simulink model "one"  (R2021a)
settings: Solver=VariableStepAuto  StartTime=0.0  StopTime=10.0  RelTol=1e-3
values from neighbouring files (symbols this model uses):
  A = eval(simplify(A))    [cfg_one.m]
  B = eval(simplify(B))    [cfg_one.m]
  K = acker(A, B, [-20 -20 -200])    [cfg_one.m]
  u_eq = double(solve(subs(fxu(1), x1, x1_eq(2))))    [cfg_one.m]
  x1_eq = double(x1_eq(2))    [cfg_one.m]
  x2_eq = 1    [cfg_one.m]
  x3_eq = 0    [cfg_one.m]
libraries: cstblocks x4
settings Model: Creator=Acer  LastModifiedBy=Acer

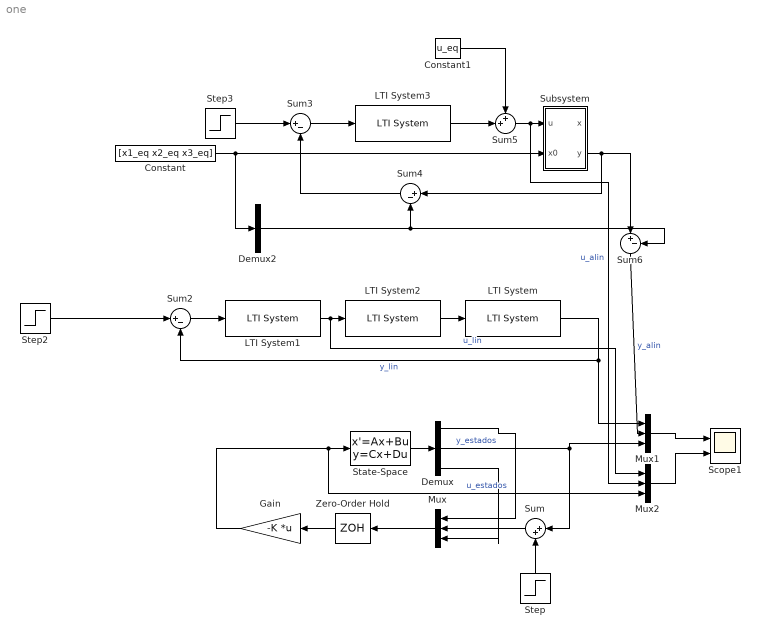
== system one ==
  Constant : Constant  Value=[x1_eq x2_eq x3_eq]
  Constant1 : Constant  Value=u_eq
  Demux : Demux  Outputs=3
  Demux2 : Demux  Outputs=3
  Gain : Gain  Gain=-K  Multiplication=Matrix(K*u) (u vector)
  LTI System : cstblocks/LTI System  sys=P  IC=[]
  LTI System1 : cstblocks/LTI System  sys=Contr  IC=[]
  LTI System2 : cstblocks/LTI System  sys=pade_raro  IC=[]
  LTI System3 : cstblocks/LTI System  sys=Contr  IC=[]
  Mux : Mux  Inputs=3
  Mux1 : Mux  Inputs=3
  Mux2 : Mux  Inputs=3
  Scope1 : Scope  NumInputPorts=2
  State-Space : StateSpace  A=A  B=B  C=eye(3)  D=zeros(3,1)  InitialCondition=0
  Step : Step  After=-0.01  SampleTime=0
  Step2 : Step  After=0.01  SampleTime=0
  Step3 : Step  After=0.01  SampleTime=0
  Subsystem : Subsystem
  Sum : Sum  Inputs=|++
  Sum{2..4,6} (4 alike) : Sum  Inputs=|+-
  Sum5 : Sum  Inputs=++|
  Zero-Order Hold : ZeroOrderHold  SampleTime=0.01/2
  wires:
  Gain/1 -> Mux2/3, State-Space/1  "u_estados"
  State-Space/1 -> Demux/1
  Demux/1 -> Mux/1
  Demux/2 -> Mux1/3, Sum/1  "y_estados"
  Demux/3 -> Mux/3
  Sum/1 -> Mux/2
  Step/1 -> Sum/2
  LTI System2/1 -> LTI System/1
  LTI System1/1 -> Mux2/1, LTI System2/1  "u_lin"
  Mux/1 -> Zero-Order Hold/1
  Zero-Order Hold/1 -> Gain/1
  LTI System/1 -> Mux1/1, Sum2/2  "y_lin"
  Sum2/1 -> LTI System1/1
  Step2/1 -> Sum2/1
  Subsystem/2(y) -> Sum6/1, Sum4/1
  Sum3/1 -> LTI System3/1
  Constant/1 -> Demux2/1, Subsystem/2(x0)
  Sum4/1 -> Sum3/2
  Demux2/2 -> Sum6/2, Sum4/2
  LTI System3/1 -> Sum5/2
  Sum5/1 -> Mux2/2, Subsystem/1(u)  "u_alin"
  Constant1/1 -> Sum5/1
  Step3/1 -> Sum3/1
  Sum6/1 -> Mux1/2  "y_alin"
  Mux1/1 -> Scope1/1
  Mux2/1 -> Scope1/2

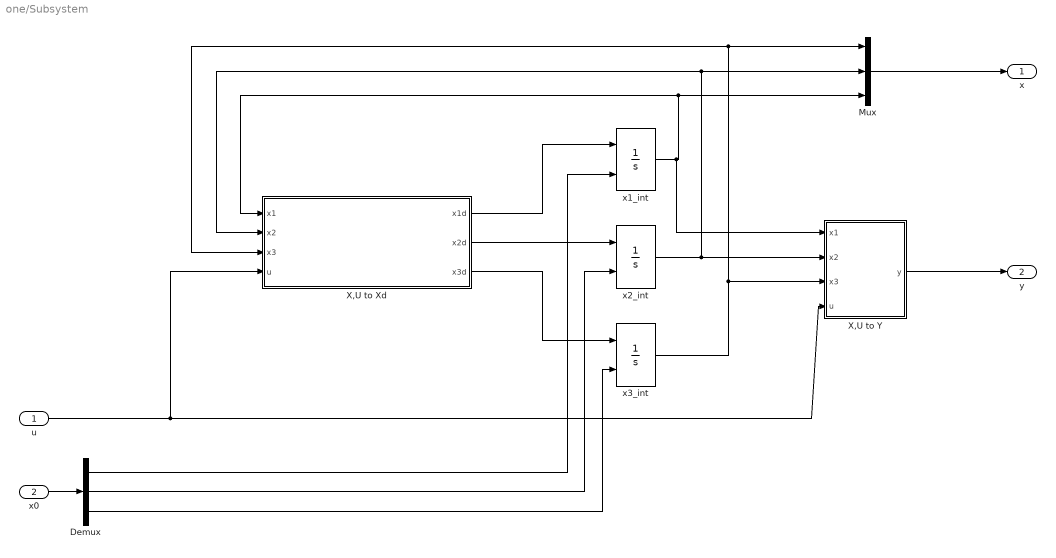
== system one/Subsystem ==
  u : Inport
  x0 : Inport  Port=2
  Demux : Demux  Outputs=3
  Mux : Mux  Inputs=3
  X,U to Xd : MATLAB Function  TreatAsAtomicUnit=on
  X,U to Y : MATLAB Function  TreatAsAtomicUnit=on
  x1_int : Integrator  InitialConditionSource=external
  x2_int : Integrator  InitialConditionSource=external
  x3_int : Integrator  InitialConditionSource=external
  x : Outport
  y : Outport  Port=2
  wires:
  x2_int/1 -> X,U to Xd/2(x2), Mux/2, X,U to Y/2(x2)
  X,U to Xd/2(x2d) -> x2_int/1
  Demux/3 -> x3_int/2
  x3_int/1 -> X,U to Xd/3(x3), Mux/1, X,U to Y/3(x3)
  u/1 -> X,U to Y/4(u), X,U to Xd/4(u)
  x1_int/1 -> X,U to Y/1(x1), Mux/3, X,U to Xd/1(x1)
  X,U to Xd/1(x1d) -> x1_int/1
  X,U to Y/1(y) -> y/1
  X,U to Xd/3(x3d) -> x3_int/1
  Demux/2 -> x2_int/2
  Mux/1 -> x/1
  x0/1 -> Demux/1
  Demux/1 -> x1_int/2

== matlab function one/Subsystem/X,U to Y ==
  data: x1 input; x2 input; x3 input; u input; y output
function y = fcn(x1,x2,x3,u)
%y = C*x+D*u
y = x2;

== matlab function one/Subsystem/X,U to Xd ==
  data: x1 input; x2 input; x3 input; u input; x1d output; x2d output; x3d output
function [x1d,x2d,x3d] = fcn(x1,x2,x3,u)

m = 1;
g = 10;
L0 = g/4;
R = 1;
L = 100e-3;
alfa = pi/4;

x1d = -x1*(R/L)+u*(1/L);
x2d = x3;
x3d = (-L0/(2*m))*(x1^2/x2^2) + g*sin(alfa);
